simulink model "fw_land_detector"  (R2024b)
settings: Solver=FixedStepAuto  StartTime=0.0  StopTime=10.0  FixedStep=0.005  RelTol=1e-3
undefined symbols (not defined in the file or in its folder): LNDFW_AIRSPD_MAX, LNDFW_VEL_XY_MAX, LNDFW_VEL_Z_MAX, LNDFW_XYACC_MAX
libraries: simulink x4
settings Model: DataDictionary=nextpilot_datadict.sldd  Creator=yu  LastModifiedBy=CETCA

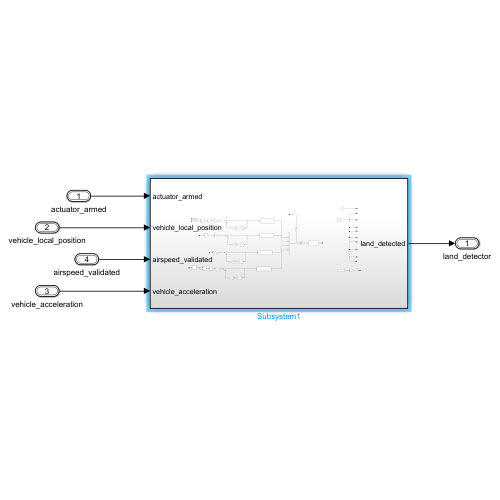
[thumbnail: Simulink's stored preview of the top-level diagram]
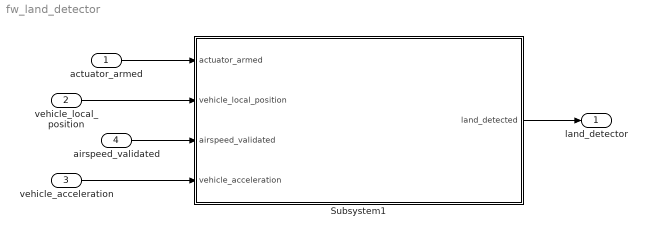
== system fw_land_detector ==
  actuator_armed : Inport  OutDataTypeStr=Bus: actuator_armed_s
  vehicle_local_position : Inport  Port=2  OutDataTypeStr=Bus: vehicle_local_position_s
  vehicle_acceleration : Inport  Port=3  OutDataTypeStr=Bus: vehicle_acceleration_s
  airspeed_validated : Inport  Port=4  OutDataTypeStr=Bus: airspeed_validated_s
  Subsystem1 : Subsystem
  land_detector : Outport  OutDataTypeStr=Bus: vehicle_land_detected_s
  wires:
  actuator_armed/1 -> Subsystem1/1(actuator_armed)
  vehicle_local_position/1 -> Subsystem1/2(vehicle_local_position)
  airspeed_validated/1 -> Subsystem1/3(airspeed_validated)
  vehicle_acceleration/1 -> Subsystem1/4(vehicle_acceleration)
  Subsystem1/1(land_detected) -> land_detector/1

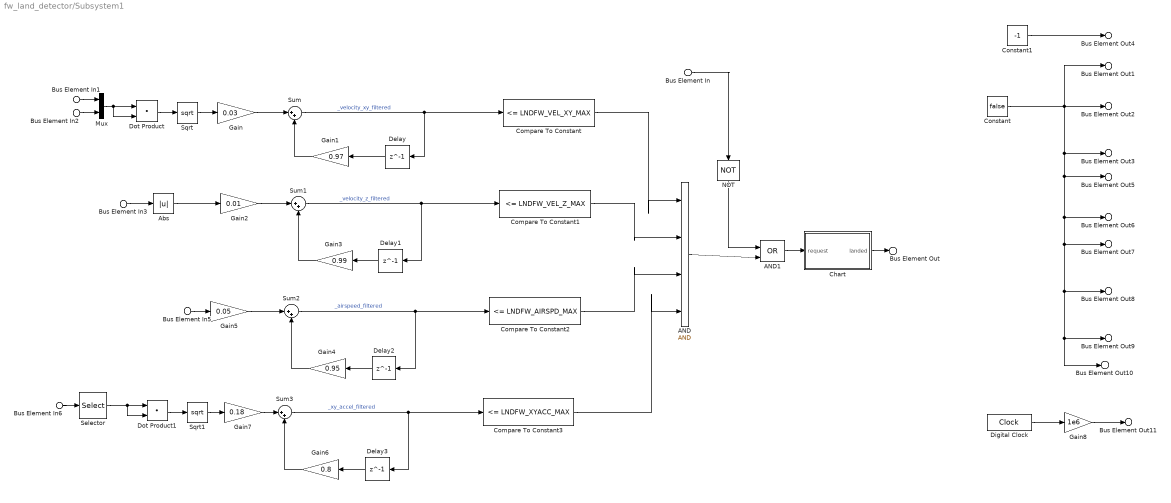
== system fw_land_detector/Subsystem1 ==
  Bus Element In : Inport  PortName=actuator_armed  Element=armed
  Bus Element In1 : Inport  Port=2  PortName=vehicle_local_position  Element=vx
  Bus Element In2 : Inport  Port=2  PortName=vehicle_local_position  Element=vy
  Bus Element In3 : Inport  Port=2  PortName=vehicle_local_position  Element=vz
  Bus Element In5 : Inport  Port=3  PortName=airspeed_validated  Element=true_airspeed_m_s
  Bus Element In6 : Inport  Port=4  PortName=vehicle_acceleration  Element=xyz
  AND : Logic  Inputs=4  IconShape=distinctive  AllPortsSameDT=off  OutDataTypeStr=boolean
  AND1 : Logic  Operator=OR  IconShape=distinctive  AllPortsSameDT=off  OutDataTypeStr=boolean
  Abs : Abs  SaturateOnIntegerOverflow=off
  Chart : Stateflow chart  TreatAsAtomicUnit=on
  Compare To Constant : simulink/Logic and Bit Operations/Compare To Constant  relop=<=  const=LNDFW_VEL_XY_MAX  OutDataTypeStr=boolean
  Compare To Constant1 : simulink/Logic and Bit Operations/Compare To Constant  relop=<=  const=LNDFW_VEL_Z_MAX  OutDataTypeStr=boolean
  Compare To Constant2 : simulink/Logic and Bit Operations/Compare To Constant  relop=<=  const=LNDFW_AIRSPD_MAX  OutDataTypeStr=boolean
  Compare To Constant3 : simulink/Logic and Bit Operations/Compare To Constant  relop=<=  const=LNDFW_XYACC_MAX  OutDataTypeStr=boolean
  Constant : Constant  Value=false
  Constant1 : Constant  Value=-1  OutDataTypeStr=single
  Delay{,1..3} (4 alike) : Delay  DelayLength=1
  Digital Clock : DigitalClock  SampleTime=-1
  Dot Product : DotProduct  OutDataTypeStr=Inherit: Inherit via internal rule
  Dot Product1 : DotProduct  OutDataTypeStr=Inherit: Inherit via internal rule
  Gain : Gain  Gain=0.03
  Gain1 : Gain  Gain=0.97
  Gain2 : Gain  Gain=0.01
  Gain3 : Gain  Gain=0.99
  Gain4 : Gain  Gain=0.95
  Gain5 : Gain  Gain=0.05
  Gain6 : Gain  Gain=0.8
  Gain7 : Gain  Gain=0.18
  Gain8 : Gain  Gain=1e6  OutDataTypeStr=uint64
  Mux : Mux  Inputs=2
  NOT : Logic  Operator=NOT  IconShape=distinctive  AllPortsSameDT=off  OutDataTypeStr=boolean
  Selector : Selector  InputPortWidth=3  IndexOptions=Index vector (dialog)  Indices=[1 2]  OutputSizes=1
  Sqrt : Sqrt
  Sqrt1 : Sqrt
  Sum{,1..3} (4 alike) : Sum  Inputs=|++
  Bus Element Out11 : Outport  PortName=land_detected  Element=timestamp
  Bus Element Out4 : Outport  PortName=land_detected  Element=alt_max
  Bus Element Out1 : Outport  PortName=land_detected  Element=freefall
  Bus Element Out3 : Outport  PortName=land_detected  Element=ground_contact
  Bus Element Out2 : Outport  PortName=land_detected  Element=maybe_landed
  Bus Element Out : Outport  PortName=land_detected  Element=landed
  Bus Element Out5 : Outport  PortName=land_detected  Element=in_ground_effect
  Bus Element Out6 : Outport  PortName=land_detected  Element=in_descend
  Bus Element Out7 : Outport  PortName=land_detected  Element=has_low_throttle
  Bus Element Out9 : Outport  PortName=land_detected  Element=vertical_movement
  Bus Element Out8 : Outport  PortName=land_detected  Element=horizontal_movement
  Bus Element Out10 : Outport  PortName=land_detected  Element=close_to_ground_or_skipped_check
  wires:
  Bus Element In2/1 -> Mux/2
  Bus Element In1/1 -> Mux/1
  Mux/1 -> Dot Product/2, Dot Product/1
  Dot Product/1 -> Sqrt/1
  Sqrt/1 -> Gain/1
  Gain/1 -> Sum/1
  Sum/1 -> Delay/1, Compare To Constant/1  "_velocity_xy_filtered"
  Delay/1 -> Gain1/1
  Gain1/1 -> Sum/2
  Bus Element In3/1 -> Abs/1
  Abs/1 -> Gain2/1
  Gain2/1 -> Sum1/1
  Sum1/1 -> Compare To Constant1/1, Delay1/1  "_velocity_z_filtered"
  Delay1/1 -> Gain3/1
  Gain3/1 -> Sum1/2
  Gain4/1 -> Sum2/2
  Delay2/1 -> Gain4/1
  Sum2/1 -> Compare To Constant2/1, Delay2/1  "_airspeed_filtered"
  Bus Element In5/1 -> Gain5/1
  Gain5/1 -> Sum2/1
  Bus Element In6/1 -> Selector/1
  Dot Product1/1 -> Sqrt1/1
  Selector/1 -> Dot Product1/2, Dot Product1/1
  Gain7/1 -> Sum3/1
  Sum3/1 -> Compare To Constant3/1, Delay3/1  "_xy_accel_filtered"
  Delay3/1 -> Gain6/1
  Gain6/1 -> Sum3/2
  Sqrt1/1 -> Gain7/1
  Compare To Constant2/1 -> AND/3
  Compare To Constant3/1 -> AND/4
  Compare To Constant1/1 -> AND/2
  Compare To Constant/1 -> AND/1
  AND/1 -> AND1/2
  Bus Element In/1 -> NOT/1
  NOT/1 -> AND1/1
  AND1/1 -> Chart/1(request)
  Constant/1 -> Bus Element Out1/1, Bus Element Out10/1, Bus Element Out9/1, Bus Element Out8/1, Bus Element Out7/1, Bus Element Out6/1, Bus Element Out5/1, Bus Element Out3/1, Bus Element Out2/1
  Digital Clock/1 -> Gain8/1
  Gain8/1 -> Bus Element Out11/1
  Constant1/1 -> Bus Element Out4/1
  Chart/1(landed) -> Bus Element Out/1

== stateflow chart fw_land_detector/Subsystem1/Chart ==
  state Landed
    en:
    landed = true;
  state Flying
    en:
    landed = false;
  (default) -> Landed : {
      | LANDED_TRIGGER_TIME_S = 2;
      | FLYING_TRIGGER_TIME_S = 0;
      | }
  Flying -> Landed : [duration(request, sec)>=LANDED_TRIGGER_TIME_S]
  Landed -> Flying : [duration(~request, sec)>=FLYING_TRIGGER_TIME_S]
  data: request input; landed output; FLYING_TRIGGER_TIME_US local; LANDED_TRIGGER_TIME_US local; LANDED_TRIGGER_TIME_S local; FLYING_TRIGGER_TIME_S local
